simulink model "Sim_exercise1"  (R2015b)
settings: Solver=VariableStepAuto  StartTime=0.0  StopTime=10.0  RelTol=1e-3
values from neighbouring files (symbols this model uses):
  A = [0 1; 0 -(dm/Jeq + Km*Kemf/(R*Jeq))]    [Exercise_3.m]
  B = [0; Km/(R*Jeq)]    [Exercise_3.m]
  C = [1/n 0; 0 1/n]    [Exercise_3.m]
  D = [0; 0]    [Exercise_3.m]
  dm = 3.8E-6    (= 3.8e-06)    [Exercise_3.m]
  Jeq = Jm + (J1+J2)/(n^2)    (= 2.186e-06)    [Exercise_3.m]
  Kemf = 137*2*pi/60    (= 14.3466064514)    [Exercise_3.m]
  Km = 69.7E-3    (= 0.0697)    [Exercise_3.m]
  L = 0    [Exercise_3.m]
  n = 5    [Exercise_3.m]
  R = 112    [Exercise_3.m]
settings Model: Creator=sofianh  LastModifiedBy=sofianh

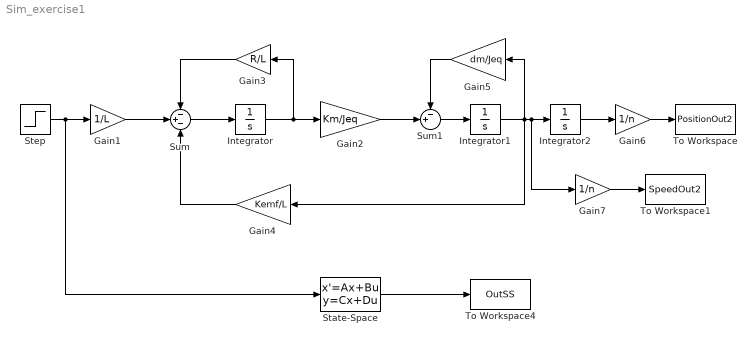
== system Sim_exercise1 ==
  Gain1 : Gain  Gain=1/L
  Gain2 : Gain  Gain=Km/Jeq
  Gain3 : Gain  Gain=R/L
  Gain4 : Gain  Gain=Kemf/L
  Gain5 : Gain  Gain=dm/Jeq
  Gain6 : Gain  Gain=1/n
  Gain7 : Gain  Gain=1/n
  Integrator : Integrator
  Integrator1 : Integrator
  Integrator2 : Integrator
  State-Space : StateSpace  A=A  B=B  C=C  D=D  X0=0  ContinuousStateAttributes='Position'
  Step : Step  Time=0  SampleTime=0
  Sum : Sum  Inputs=-+-
  Sum1 : Sum  Inputs=-+|
  To Workspace : ToWorkspace  VariableName=PositionOut2  SaveFormat=Structure With Time  SampleTime=-1
  To Workspace1 : ToWorkspace  VariableName=SpeedOut2  SaveFormat=Structure With Time  SampleTime=-1
  To Workspace4 : ToWorkspace  VariableName=OutSS  SaveFormat=Structure With Time  SampleTime=-1
  wires:
  State-Space/1 -> To Workspace4/1
  Step/1 -> State-Space/1, Gain1/1
  Gain1/1 -> Sum/2
  Sum/1 -> Integrator/1
  Integrator/1 -> Gain3/1, Gain2/1
  Sum1/1 -> Integrator1/1
  Gain2/1 -> Sum1/2
  Integrator1/1 -> Gain5/1, Gain4/1, Gain7/1, Integrator2/1
  Gain3/1 -> Sum/1
  Gain4/1 -> Sum/3
  Gain5/1 -> Sum1/1
  Integrator2/1 -> Gain6/1
  Gain6/1 -> To Workspace/1
  Gain7/1 -> To Workspace1/1
